simulink model "mcb_host_common"  (R2022a)
settings: Solver=FixedStepDiscrete  StartTime=0.0  StopTime=inf  RelTol=1e-3  EnableMultiTasking=on
undefined symbols (not defined in the file): PU_System
libraries: instrumentseriallib x4, simulink x2
settings Model: Creator=The MathWorks, Inc.  LastModifiedBy=I52209
settings SolverCC: AlgebraicLoopSolver=TrustRegion
settings DataIOCC: LimitDataPoints=on  SaveFormat=Array  ReturnWorkspaceOutputs=off
settings OptimizationCC: LifeSpan=1  EfficientTunableParamExpr=on
settings DebuggingCC: MergeDetectMultiDrivingBlocksExec=none  SolverPrmCheckMsg=warning  ParameterPrecisionLossMsg=none  UnconnectedInputMsg=warning  UnconnectedOutputMsg=warning  UnconnectedLineMsg=warning  AllowSymbolicDim=off  PregeneratedLibrarySubsystemCodeDiagnostic=none  SFUnexpectedBacktrackingDiag=warning  SFNoUnconditionalDefaultTransitionDiag=warning  SFExecutionAtInitializationDiag=none  SFMachineParentedDataDiag=warning  ArithmeticOperatorsInVariantConditions=warning
settings HardwareCC: ProdBitPerPointer=32  ProdLargestAtomicFloat=None  ProdIntDivRoundTo=Undefined  ProdEndianess=Unspecified  ProdWordSize=32  ProdHWDeviceType=32-bit Generic
settings ModelReferenceCC: PropagateSignalLabelsOutOfModel=off
settings SFSimCC: SimUseLocalCustomCode=off  MATLABDynamicMemAlloc=off
settings RTWCC: Description=Real-Time Workshop Embedded Coder  SystemTargetFile=ert.tlc  TemplateMakefile=ert_default_tmf  GenerateReport=on  RTWUseLocalCustomCode=off  IncludeHyperlinkInReport=on  LaunchReport=on  GenerateTraceInfo=on  GenerateTraceReport=on  GenerateTraceReportSl=on  GenerateTraceReportSf=on  GenerateTraceReportEml=on  DLArmComputeVersion=19.05
settings CodeAppCC: IgnoreCustomStorageClasses=off  StateflowObjectComments=on  InternalIdentifier=Classic
settings ERTTargetCC: MultiwordLength=2048  GenerateSampleERTMain=on  ERTCustomFileTemplate=example_file_process.tlc  ConvertIfToSwitch=off  SuppressUnreachableDefaultCases=off
settings ConfigComp: CovMetricSettings=dw  CovSaveCumulativeToWorkspaceVar=on  CovSaveSingleToWorkspaceVar=on  CovExternalEMLEnable=off  CovSFcnEnable=off

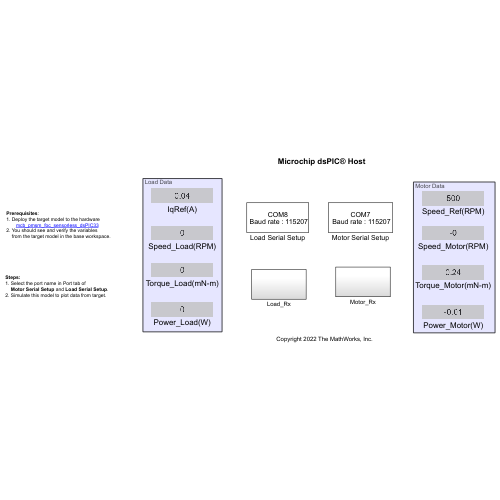
[thumbnail: Simulink's stored preview of the top-level diagram]
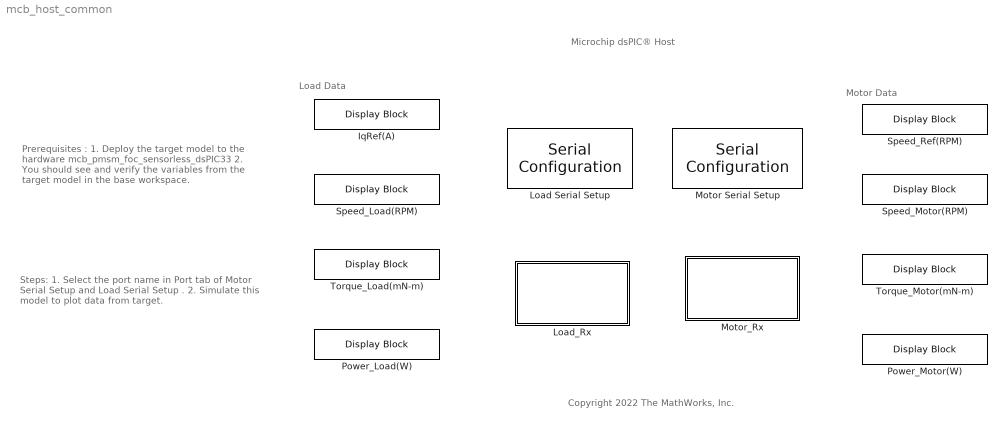
== system mcb_host_common ==
  note: Load Data
  note: Motor Data
  note: Steps:
      | 1. Select the port name in Port tab of
      | Motor Serial Setup and Load Serial Setup .
      | 2. Simulate this model to plot data from target.
  note: Prerequisites :
      | 1. Deploy the target model to the hardware
      | mcb_pmsm_foc_sensorless_dsPIC33
      | 2. You should see and verify the variables
      | from the target model in the base workspace.
  note: Microchip dsPIC® Host
  note: Copyright 2022 The MathWorks, Inc.
  IqRef(A) : DisplayBlock  LabelPosition=Hide  Format=bank  Transparency=1
  Load Serial Setup : instrumentseriallib/Serial Configuration  Priority=-99  PortSel=COM8  Port=COM8  ComPort=COM8  BaudRate=115207  DataBits=8  Parity=none  StopBits=1  ByteOrder=little-endian  FlowControl=none  Timeout=2  SimulateUsing=Interpreted execution  BlockInModel=on  aMode=5
      settings: SourceProductBaseCode=OT,IC,MT
  Load_Rx : Subsystem
  Motor Serial Setup : instrumentseriallib/Serial Configuration  Priority=-99  PortSel=COM7  Port=COM7  ComPort=COM7  BaudRate=115207  DataBits=8  Parity=none  StopBits=1  ByteOrder=little-endian  FlowControl=none  Timeout=2  SimulateUsing=Interpreted execution  BlockInModel=on  aMode=5
      settings: SourceProductBaseCode=OT,IC,MT
  Motor_Rx : Subsystem
  Power_Load(W) : DisplayBlock  LabelPosition=Hide  Format=bank  Transparency=1
  Power_Motor(W) : DisplayBlock  LabelPosition=Hide  Format=bank  Transparency=1  FormatString=%i
  Speed_Load(RPM) : DisplayBlock  LabelPosition=Hide  Format=Integer  Transparency=1
  Speed_Motor(RPM) : DisplayBlock  LabelPosition=Hide  Format=Integer  Transparency=1
  Speed_Ref(RPM) : DisplayBlock  LabelPosition=Hide  Format=Integer  Transparency=1
  Torque_Load(mN-m) : DisplayBlock  LabelPosition=Hide  Format=bank  Transparency=1
  Torque_Motor(mN-m) : DisplayBlock  LabelPosition=Hide  Format=bank  Transparency=1

== system mcb_host_common/Load_Rx ==
  note: RX
  Debug Data : Subsystem
  Demux : Demux  Outputs=3
  Host Serial Receive : instrumentseriallib/Serial Receive  PortSel=COM8  Port=COM8  ComPort=COM8  DataType=uint8  SaveDataType=uint8  ToggleHeader=on  Header='S'  ToggleTerminator=on  Terminator=Custom terminator  CustomTerminator='E'  InputFormat=Row major  ToggleDataSize=on  DataSize=3  EnableBlockingMode=on  ActionDataUnavailable=Output custom value  ActionWhenDataUnavailable=Output custom value  CustomValue=15  SampleTime=0.1  SimulateUsing=Interpreted execution  BlockInModel=on  aMode=5
      settings: SourceProductBaseCode=OT,IC,MT
  wires:
  Demux/3 -> Debug Data/3(Output3)
  Demux/2 -> Debug Data/2(Output2)
  Demux/1 -> Debug Data/1(Output1)
  Host Serial Receive/1 -> Demux/1

== system mcb_host_common/Motor_Rx ==
  note: RX
  Debug Data : Subsystem
  Demux : Demux  Outputs=3
  Host Serial Receive : instrumentseriallib/Serial Receive  PortSel=COM7  Port=COM7  ComPort=COM7  DataType=uint8  SaveDataType=uint8  ToggleHeader=on  Header='S'  ToggleTerminator=on  Terminator=Custom terminator  CustomTerminator='E'  InputFormat=Row major  ToggleDataSize=on  DataSize=3  EnableBlockingMode=on  ActionDataUnavailable=Output custom value  ActionWhenDataUnavailable=Output custom value  CustomValue=15  SampleTime=0.1  SimulateUsing=Interpreted execution  BlockInModel=on  aMode=5
      settings: SourceProductBaseCode=OT,IC,MT
  wires:
  Host Serial Receive/1 -> Demux/1
  Demux/1 -> Debug Data/1(Output1)
  Demux/2 -> Debug Data/2(Output2)
  Demux/3 -> Debug Data/3(Output3)

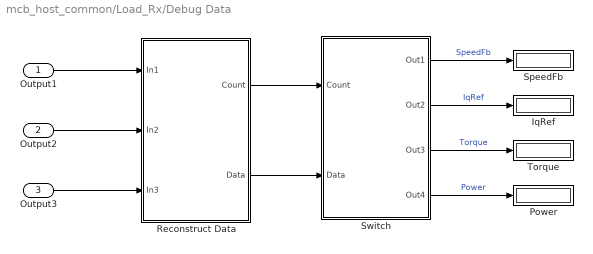
== system mcb_host_common/Load_Rx/Debug Data ==
  Output1 : Inport
  Output2 : Inport  Port=2
  Output3 : Inport  Port=3
  IqRef : Display
  Power : Display
  Reconstruct Data : Subsystem
  SpeedFb : Display
  Switch : Subsystem
  Torque : Display
  wires:
  Switch/4(Out4) -> Power/1  "Power"
  Switch/3(Out3) -> Torque/1  "Torque"
  Switch/2(Out2) -> IqRef/1  "IqRef"
  Switch/1(Out1) -> SpeedFb/1  "SpeedFb"
  Reconstruct Data/2(Data) -> Switch/2(Data)
  Reconstruct Data/1(Count) -> Switch/1(Count)
  Output3/1 -> Reconstruct Data/3(In3)
  Output2/1 -> Reconstruct Data/2(In2)
  Output1/1 -> Reconstruct Data/1(In1)

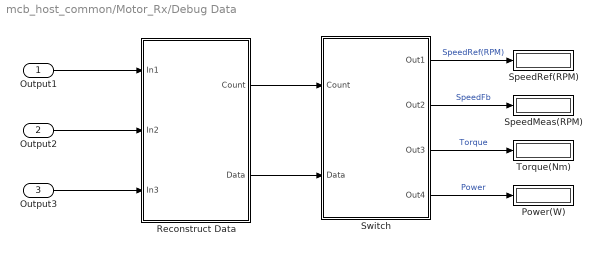
== system mcb_host_common/Motor_Rx/Debug Data ==
  Output1 : Inport
  Output2 : Inport  Port=2
  Output3 : Inport  Port=3
  Power(W) : Display
  Reconstruct Data : Subsystem
  SpeedMeas(RPM) : Display
  SpeedRef(RPM) : Display
  Switch : Subsystem
  Torque(Nm) : Display
  wires:
  Output1/1 -> Reconstruct Data/1(In1)
  Output2/1 -> Reconstruct Data/2(In2)
  Output3/1 -> Reconstruct Data/3(In3)
  Reconstruct Data/1(Count) -> Switch/1(Count)
  Reconstruct Data/2(Data) -> Switch/2(Data)
  Switch/1(Out1) -> SpeedRef(RPM)/1  "SpeedRef(RPM)"
  Switch/2(Out2) -> SpeedMeas(RPM)/1  "SpeedFb"
  Switch/3(Out3) -> Torque(Nm)/1  "Torque"
  Switch/4(Out4) -> Power(W)/1  "Power"

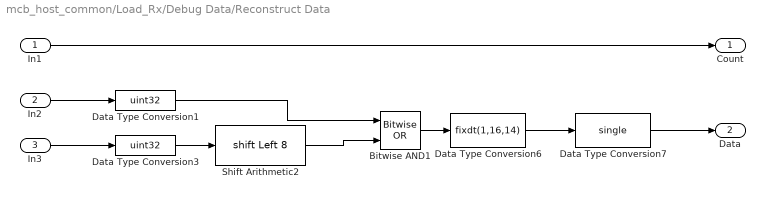
== system mcb_host_common/Load_Rx/Debug Data/Reconstruct Data ==
  In1 : Inport
  In2 : Inport  Port=2
  In3 : Inport  Port=3
  Bitwise AND1 : simulink/Logic and Bit Operations/Bitwise Operator  logicop=OR  UseBitMask=off  NumInputPorts=2  BitMask=bin2dec('11011001')  BitMaskRealWorld=Stored Integer
  Data Type Conversion1 : DataTypeConversion  OutDataTypeStr=uint32  RndMeth=Simplest  SaturateOnIntegerOverflow=off
  Data Type Conversion3 : DataTypeConversion  OutDataTypeStr=uint32  RndMeth=Simplest  SaturateOnIntegerOverflow=off
  Data Type Conversion6 : DataTypeConversion  OutDataTypeStr=fixdt(1,16,14)  ConvertRealWorld=Stored Integer (SI)  RndMeth=Simplest  SaturateOnIntegerOverflow=off
  Data Type Conversion7 : DataTypeConversion  OutDataTypeStr=single  RndMeth=Simplest  SaturateOnIntegerOverflow=off
  Shift Arithmetic2 : ArithShift  BitShiftNumber=8  BitShiftDirection=Left
  Count : Outport
  Data : Outport  Port=2
  wires:
  In3/1 -> Data Type Conversion3/1
  In2/1 -> Data Type Conversion1/1
  In1/1 -> Count/1
  Data Type Conversion7/1 -> Data/1
  Data Type Conversion1/1 -> Bitwise AND1/1
  Data Type Conversion3/1 -> Shift Arithmetic2/1
  Bitwise AND1/1 -> Data Type Conversion6/1
  Data Type Conversion6/1 -> Data Type Conversion7/1
  Shift Arithmetic2/1 -> Bitwise AND1/2

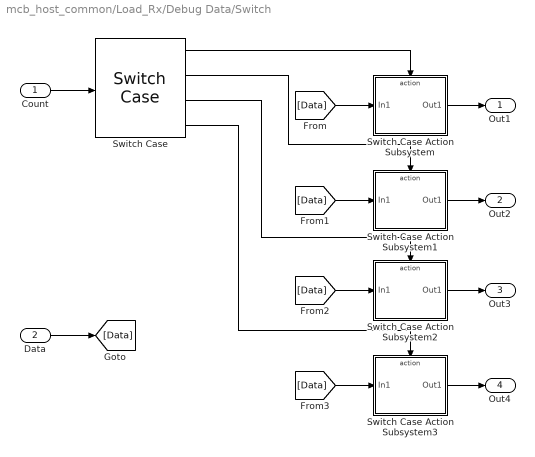
== system mcb_host_common/Load_Rx/Debug Data/Switch ==
  Count : Inport
  Data : Inport  Port=2
  Switch Case : SwitchCase  CaseConditions={0,1,2,3}  ShowDefaultCase=off
  Switch Case Action Subsystem : Subsystem  TreatAsAtomicUnit=on
  Switch Case Action Subsystem1 : Subsystem  TreatAsAtomicUnit=on
  Switch Case Action Subsystem2 : Subsystem  TreatAsAtomicUnit=on
  Switch Case Action Subsystem3 : Subsystem  TreatAsAtomicUnit=on
  Out1 : Outport
  Out2 : Outport  Port=2
  Out3 : Outport  Port=3
  Out4 : Outport  Port=4
  wires:
  [Data] -> Switch Case Action Subsystem/1(In1)
  Switch Case Action Subsystem/1(Out1) -> Out1/1
  Switch Case/2 -> Switch Case Action Subsystem1/Action
  [Data] -> Switch Case Action Subsystem1/1(In1)
  Switch Case/3 -> Switch Case Action Subsystem2/Action
  Switch Case/4 -> Switch Case Action Subsystem3/Action
  Data/1 -> [Data]
  Count/1 -> Switch Case/1
  [Data] -> Switch Case Action Subsystem2/1(In1)
  Switch Case Action Subsystem2/1(Out1) -> Out3/1
  Switch Case Action Subsystem1/1(Out1) -> Out2/1
  Switch Case Action Subsystem3/1(Out1) -> Out4/1
  [Data] -> Switch Case Action Subsystem3/1(In1)
  Switch Case/1 -> Switch Case Action Subsystem/Action

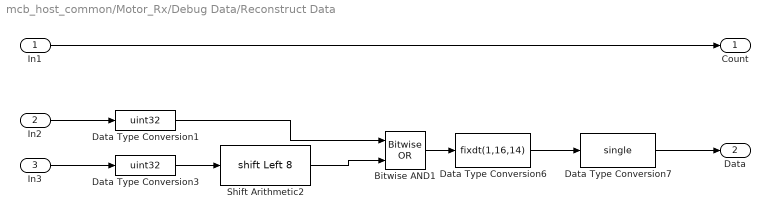
== system mcb_host_common/Motor_Rx/Debug Data/Reconstruct Data ==
  In1 : Inport
  In2 : Inport  Port=2
  In3 : Inport  Port=3
  Bitwise AND1 : simulink/Logic and Bit Operations/Bitwise Operator  logicop=OR  UseBitMask=off  NumInputPorts=2  BitMask=bin2dec('11011001')  BitMaskRealWorld=Stored Integer
  Data Type Conversion1 : DataTypeConversion  OutDataTypeStr=uint32  RndMeth=Simplest  SaturateOnIntegerOverflow=off
  Data Type Conversion3 : DataTypeConversion  OutDataTypeStr=uint32  RndMeth=Simplest  SaturateOnIntegerOverflow=off
  Data Type Conversion6 : DataTypeConversion  OutDataTypeStr=fixdt(1,16,14)  ConvertRealWorld=Stored Integer (SI)  RndMeth=Simplest  SaturateOnIntegerOverflow=off
  Data Type Conversion7 : DataTypeConversion  OutDataTypeStr=single  RndMeth=Simplest  SaturateOnIntegerOverflow=off
  Shift Arithmetic2 : ArithShift  BitShiftNumber=8  BitShiftDirection=Left
  Count : Outport
  Data : Outport  Port=2
  wires:
  Shift Arithmetic2/1 -> Bitwise AND1/2
  Data Type Conversion6/1 -> Data Type Conversion7/1
  Bitwise AND1/1 -> Data Type Conversion6/1
  Data Type Conversion3/1 -> Shift Arithmetic2/1
  Data Type Conversion1/1 -> Bitwise AND1/1
  Data Type Conversion7/1 -> Data/1
  In2/1 -> Data Type Conversion1/1
  In3/1 -> Data Type Conversion3/1
  In1/1 -> Count/1

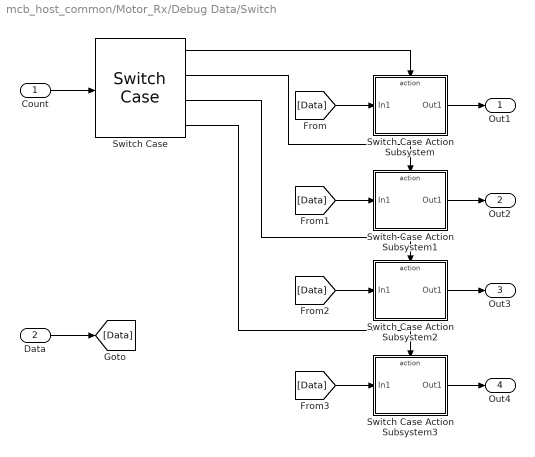
== system mcb_host_common/Motor_Rx/Debug Data/Switch ==
  Count : Inport
  Data : Inport  Port=2
  Switch Case : SwitchCase  CaseConditions={0,1,2,3}  ShowDefaultCase=off
  Switch Case Action Subsystem : Subsystem  TreatAsAtomicUnit=on
  Switch Case Action Subsystem1 : Subsystem  TreatAsAtomicUnit=on
  Switch Case Action Subsystem2 : Subsystem  TreatAsAtomicUnit=on
  Switch Case Action Subsystem3 : Subsystem  TreatAsAtomicUnit=on
  Out1 : Outport
  Out2 : Outport  Port=2
  Out3 : Outport  Port=3
  Out4 : Outport  Port=4
  wires:
  Switch Case/1 -> Switch Case Action Subsystem/Action
  [Data] -> Switch Case Action Subsystem3/1(In1)
  Switch Case Action Subsystem3/1(Out1) -> Out4/1
  Switch Case Action Subsystem1/1(Out1) -> Out2/1
  Switch Case Action Subsystem2/1(Out1) -> Out3/1
  [Data] -> Switch Case Action Subsystem2/1(In1)
  Count/1 -> Switch Case/1
  Data/1 -> [Data]
  Switch Case/4 -> Switch Case Action Subsystem3/Action
  Switch Case/3 -> Switch Case Action Subsystem2/Action
  [Data] -> Switch Case Action Subsystem1/1(In1)
  Switch Case/2 -> Switch Case Action Subsystem1/Action
  Switch Case Action Subsystem/1(Out1) -> Out1/1
  [Data] -> Switch Case Action Subsystem/1(In1)

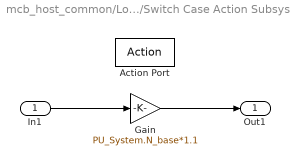
== system mcb_host_common/Load_Rx/Debug Data/Switch/Switch Case Action Subsystem ==
  In1 : Inport
  Action Port : ActionPort  ActionPortLabel=case [ 0 ]:
  Gain : Gain  Gain=PU_System.N_base*1.1
  Out1 : Outport
  wires:
  In1/1 -> Gain/1
  Gain/1 -> Out1/1

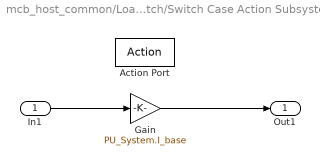
== system mcb_host_common/Load_Rx/Debug Data/Switch/Switch Case Action Subsystem1 ==
  In1 : Inport
  Action Port : ActionPort  ActionPortLabel=case [ 1 ]:
  Gain : Gain  Gain=PU_System.I_base
  Out1 : Outport
  wires:
  Gain/1 -> Out1/1
  In1/1 -> Gain/1

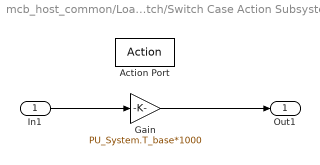
== system mcb_host_common/Load_Rx/Debug Data/Switch/Switch Case Action Subsystem2 ==
  In1 : Inport
  Action Port : ActionPort  ActionPortLabel=case [ 2 ]:
  Gain : Gain  Gain=PU_System.T_base*1000
  Out1 : Outport
  wires:
  Gain/1 -> Out1/1
  In1/1 -> Gain/1

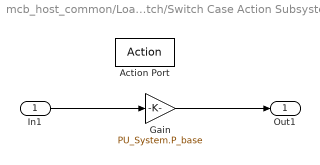
== system mcb_host_common/Load_Rx/Debug Data/Switch/Switch Case Action Subsystem3 ==
  In1 : Inport
  Action Port : ActionPort  ActionPortLabel=case [ 3 ]:
  Gain : Gain  Gain=PU_System.P_base
  Out1 : Outport
  wires:
  Gain/1 -> Out1/1
  In1/1 -> Gain/1

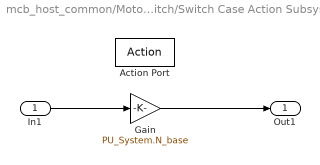
== system mcb_host_common/Motor_Rx/Debug Data/Switch/Switch Case Action Subsystem ==
  In1 : Inport
  Action Port : ActionPort  ActionPortLabel=case [ 0 ]:
  Gain : Gain  Gain=PU_System.N_base
  Out1 : Outport
  wires:
  In1/1 -> Gain/1
  Gain/1 -> Out1/1

== system mcb_host_common/Motor_Rx/Debug Data/Switch/Switch Case Action Subsystem1 ==
  In1 : Inport
  Action Port : ActionPort  ActionPortLabel=case [ 1 ]:
  Gain : Gain  Gain=PU_System.N_base
  Out1 : Outport
  wires:
  In1/1 -> Gain/1
  Gain/1 -> Out1/1

== system mcb_host_common/Motor_Rx/Debug Data/Switch/Switch Case Action Subsystem2 ==
  In1 : Inport
  Action Port : ActionPort  ActionPortLabel=case [ 2 ]:
  Gain : Gain  Gain=PU_System.T_base*1000
  Out1 : Outport
  wires:
  In1/1 -> Gain/1
  Gain/1 -> Out1/1

== system mcb_host_common/Motor_Rx/Debug Data/Switch/Switch Case Action Subsystem3 ==
  In1 : Inport
  Action Port : ActionPort  ActionPortLabel=case [ 3 ]:
  Gain : Gain  Gain=PU_System.P_base
  Out1 : Outport
  wires:
  In1/1 -> Gain/1
  Gain/1 -> Out1/1
